simulink subsystem "ConfiguredSimscapePlantModels"  (R2022b)
settings: Solver=VariableStepAuto  StartTime=0.0  StopTime=10.0  RelTol=1e-3
undefined symbols (not defined in the file): AxlFL, AxlFR, AxlRL, AxlRR, EM1, EM2, PlntDCDCVoltInit, PlntDiffrntl2Axl1Damp, PlntDiffrntl2CarrDamp, PlntDiffrntl2Eff, PlntDiffrntl2PwrThresh, PlntDiffrntlAxl1Damp, PlntDiffrntlCarrDamp, PlntDiffrntlEff, PlntDiffrntlPwrThresh, PlntTrnsfrCaseAxlSpdLock, PlntTrnsfrCaseTrqSplitRatio
libraries: fl_lib x14, nesl_utility_internal x10, sdl_lib x5, nesl_utility x1
(part 2 of 2)

== system ConfiguredSimscapePlantModels/Drivetrain/Drivetrain Layout/Front Axle/Open Differential with Loss ==
  note: Copyright 2022 The MathWorks, Inc.
  DiffLoss : Subsystem  ReferencedSubsystem=DiffLoss
  DiffLoss1 : Subsystem  ReferencedSubsystem=DiffLoss
  Open Differential : sdl_lib/Gears/Differential  driveshaft_location=sdl.enum.differential_orientation.right  cd_ratio=PlntDiffrntlRatio  friction_model=sdl.enum.gear_friction.constant  efficiency=[PlntDiffrntlEff PlntDiffrntlEff]  temperature_TLU=[280, 300, 320] K  efficiency_ss_TLU=[.95, .9, .85]  efficiency_cd_TLU=[.95, .9, .85]  pwr_thr=[PlntDiffrntlPwrThresh, PlntDiffrntlPwrThresh] W  mu_visc=[PlntDiffrntlCarrDamp PlntDiffrntlAxl1Damp] N*m*s/rad  model_inertia=simscape.enum.onoff.off  carrier_inertia=PlntDiffrntlCarrInertia kg*m^2  planet_inertia=PlntDiffrntlAxl1Inertia kg*m^2  thermal_mass=50 J/K  T_init=300 K
  DriveshftTrq : PMIOPort  Side=Left
  AxlTrqFR : PMIOPort  Port=2  Side=Right
  AxlTrqFL : PMIOPort  Port=3  Side=Right
  connections:
  DiffLoss1/LConn1 -- Open Differential/RConn2
  Open Differential/LConn1 -- DriveshftTrq/RConn1
  DiffLoss1/RConn1 -- AxlTrqFR/RConn1
  AxlTrqFL/RConn1 -- DiffLoss/RConn1
  DiffLoss/LConn1 -- Open Differential/RConn1

== system ConfiguredSimscapePlantModels/Drivetrain/Drivetrain Layout/Rear Axle/Open Differential with loss ==
  note: Copyright 2022 The MathWorks, Inc.
  DiffLoss : Subsystem  ReferencedSubsystem=DiffLoss
  DiffLoss1 : Subsystem  ReferencedSubsystem=DiffLoss
  Open Differential : sdl_lib/Gears/Differential  driveshaft_location=sdl.enum.differential_orientation.right  cd_ratio=PlntDiffrntl2Ratio  friction_model=sdl.enum.gear_friction.constant  efficiency=[PlntDiffrntl2Eff PlntDiffrntl2Eff]  temperature_TLU=[280, 300, 320] K  efficiency_ss_TLU=[.95, .9, .85]  efficiency_cd_TLU=[.95, .9, .85]  pwr_thr=[PlntDiffrntl2PwrThresh, PlntDiffrntl2PwrThresh] W  mu_visc=[PlntDiffrntl2CarrDamp PlntDiffrntl2Axl1Damp] N*m*s/rad  model_inertia=simscape.enum.onoff.off  carrier_inertia=PlntDiffrntl2CarrInertia kg*m^2  planet_inertia=PlntDiffrntl2Axl1Inertia kg*m^2  thermal_mass=50 J/K  T_init=300 K
  DriveshftTrq : PMIOPort  Side=Left
  AxlTrqRR : PMIOPort  Port=2  Side=Right
  AxlTrqRL : PMIOPort  Port=3  Side=Right
  connections:
  DiffLoss/LConn1 -- Open Differential/RConn1
  DiffLoss1/LConn1 -- Open Differential/RConn2
  Open Differential/LConn1 -- DriveshftTrq/RConn1
  DiffLoss/RConn1 -- AxlTrqRL/RConn1
  DiffLoss1/RConn1 -- AxlTrqRR/RConn1

== system ConfiguredSimscapePlantModels/Electrical System/Electrical System 1EM/DC-DC Converter/No DC-DC Converter ==
  1+ : PMIOPort  Side=Left
  1- : PMIOPort  Port=2  Side=Left
  2+ : PMIOPort  Port=3  Side=Right
  2- : PMIOPort  Port=4  Side=Right
  connections:
  1-/RConn1 -- 2-/RConn1
  1+/RConn1 -- 2+/RConn1
